simulink model "FinalProject"  (R2022b)
settings: Solver=VariableStepAuto  StartTime=0.0  StopTime=800  RelTol=1e-3
InitFcn:
  | vehicle_longitudinal_para
values from neighbouring files (symbols this model uses):
  A = [-1/(R2*C2), 0; 0, 0]    [vehicle_longitudinal_para.m]
  ai = [0.0059 0.0049 0.0039 0.0028 0.0036 0.006 0.0082 0.008 0.009 0.0099]    [vehicle_longitudinal_para.m]
  B = [1/C2; ni/Cn]    [vehicle_longitudinal_para.m]
  BatteryCapacity = 10080    [vehicle_longitudinal_para.m]
  bi = [3.5052 3.5188 3.5397 3.5728 3.5416 3.4199 3.2864 3.3004 3.2232 3.1364]    [vehicle_longitudinal_para.m]
  bp = [0.05 0.15 0.25 0.35 0.45 0.55 0.65 0.75 0.85 0.95]    [vehicle_longitudinal_para.m]
  capacity = 84    [vehicle_longitudinal_para.m]
  Cr = 0.0085    [VehicleLongtitudinalModel.m]    (also in vehicle_longitudinal_para.m = 0.009)
  D = R1    (= 0.0027)    [vehicle_longitudinal_para.m]
  eng_consum_fuel = [0 0 0 0 0 0 0 0 0 0 0 0 ... (1220 elements, 61x20)]    [eng_consum_fuel.mat]    (also in vehicle_longitudinal_para.m = eng_consum_fuel * 6)
  eng_consum_spd = [52.35 55 57.6 60.2 62.85 65.45 68.05 70.7 73.3 75.9 78.55 81.15 ... (61 elements, 1x61)]    [eng_consum_fuel.mat]    (also in vehicle_longitudinal_para.m = eng_consum_spd / 2)
  eng_consum_trq = [0 137.659783677 206.489675516 275.319567355 344.149459194 412.979351032 481.809242871 550.63913471 619.469026549 688.298918387 757.128810226 825.958702065 ... (20 elements, 1x20)]    [eng_consum_fuel.mat]    (also in vehicle_longitudinal_para.m = eng_consum_trq * (1400 / 1.356 / 75))
  FD_ratio = 4.56    [vehicle_longitudinal_para.m]
  g = 9.81    [VehicleLongtitudinalModel.m]    (also in vehicle_longitudinal_para.m)
  m_map_spd = [0 52.3598775598 104.71975512 157.079632679 209.439510239 261.799387799 314.159265359 366.519142919 418.879020479 471.238898038 628.318530718]    [m_eff_map.mat]    (also in vehicle_longitudinal_para.m = [0 500 1000 1500 2000 2500 3000 3500 4000 4500 6000]*(2*pi)/)
  m_max_trq = interp1(m_spd_data,m_max_trq_data,m_map_spd,'linear')    [vehicle_longitudinal_para.m]
  P_demand = [0 22222.2222222 44444.4444444 66666.6666667 88888.8888889 111111.111111 133333.333333 155555.555556 177777.777778 200000]    [ecms_lookup.mat]    (also in ecms_model.m = linspace(0,Pmax,10); vehicle_longitudinal_para.m = linspace(0,Pmax,10))
  P_eng_opt = [0 0 0 0 0 0 0 0 0 0 0 0 ... (1100 elements, 10x10x11)]    [ecms_lookup.mat]    (also in ecms_model.m = zeros(length(P_demand),length(V_range),length(SOC_range)); vehicle_longitudinal_para.m = zeros(length(P_demand),length(V_range),length(SOC_range)))
  R_tire = 0.5    [VehicleLongtitudinalModel.m]    (also in vehicle_longitudinal_para.m = 0.74)
  SOC = [0 20 40 60 80 100]    [vehicle_longitudinal_para.m]
  SOC_H = 1.0    (= 1)    [ecms_model.m]    (also in vehicle_longitudinal_para.m = 0.9)
  SOC_L = 0.2    [ecms_model.m]    (also in vehicle_longitudinal_para.m = 0.1)
  SOC_range = [0 0.1 0.2 0.3 0.4 0.5 0.6 0.7 0.8 0.9 1]    [ecms_lookup.mat]    (also in ecms_model.m = 0:.1:1; vehicle_longitudinal_para.m = 0:.1:1)
  Speed = cdata{2}    [vehicle_longitudinal_para.m]
  testTime = [0, 1, 2, 3, 4, 5, 6, 7, 8, 9]    [vehicle_longitudinal_para.m]
  Time = cdata{1}    [vehicle_longitudinal_para.m]
  V_range = [0 23.2710566933 46.5421133865 69.8131700798 93.084226773 116.355283466 139.62634016 162.897396853 186.168453546 209.439510239]    [ecms_lookup.mat]    (also in ecms_model.m = linspace(0,Vmax,10)*2*pi/60; vehicle_longitudinal_para.m = linspace(0,Vmax,10)*2*pi/60)
  Vehicle_mass = 15076    [VehicleLongtitudinalModel.m]    (also in vehicle_longitudinal_para.m = 6273)
  weightfactor = [1 1 1 1 1 0]    [vehicle_longitudinal_para.m]
  weightfactor_ws = [0.01 0.01 1 1 1]    [vehicle_longitudinal_para.m]
  WheelSpeed = [0 30 100 150 201]    [vehicle_longitudinal_para.m]
libraries: slpidlib x2
settings Model: Creator=12159  LastModifiedBy=12159
settings SolverCC: ZeroCrossAlgorithm=Adaptive
settings DebuggingCC: IgnoredZcDiagnostic=none

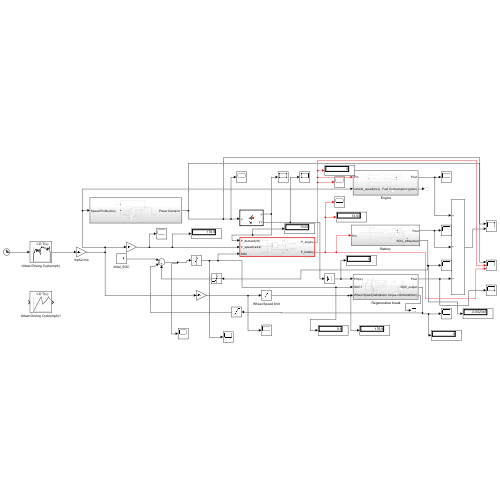
[thumbnail: Simulink's stored preview of the top-level diagram]
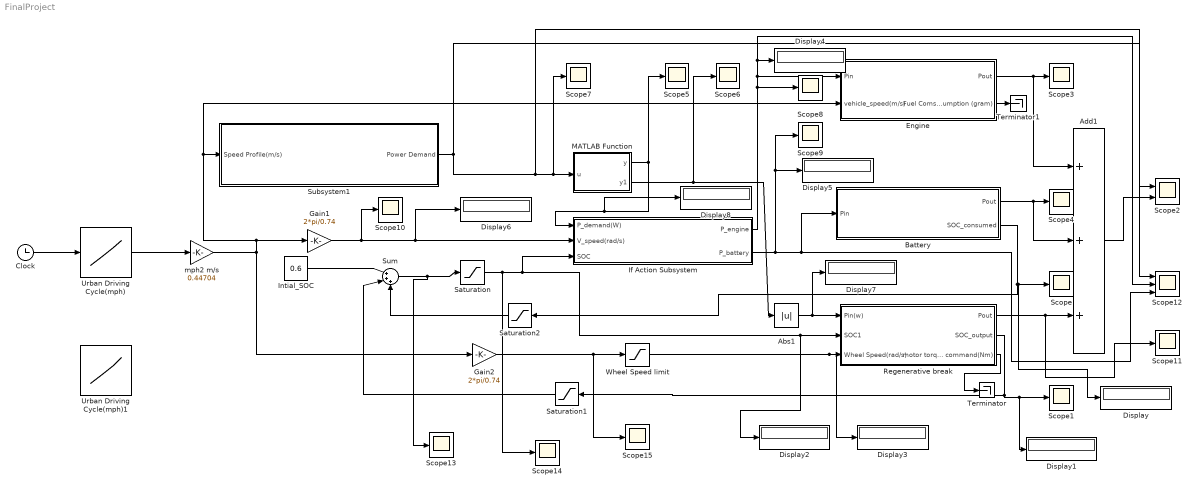
== system FinalProject ==
  " Engine" : Subsystem
  " Regenerative break" : Subsystem
  Abs1 : Abs  SaturateOnIntegerOverflow=off
  Add1 : Sum  Inputs=3
  Battery : Subsystem
  Clock : Clock
  Display{,1..8} (9 alike) : Display
  Gain1 : Gain  Gain=2*pi/0.74
  Gain2 : Gain  Gain=2*pi/0.74
  If Action Subsystem : Subsystem  TreatAsAtomicUnit=on
  Intial_SOC : Constant  Value=0.6
  MATLAB Function : MATLAB Function  TreatAsAtomicUnit=on
  Saturation : Saturate  UpperLimit=SOC_H  LowerLimit=SOC_L
  Saturation1 : Saturate  UpperLimit=SOC_H  LowerLimit=SOC_L
  Saturation2 : Saturate  UpperLimit=SOC_H  LowerLimit=SOC_L
  Scope{,1,3..11,13..15} (14 alike) : Scope
  Scope12 : Scope  NumInputPorts=3
  Scope2 : Scope  NumInputPorts=2
  Subsystem1 : Subsystem
  Sum : Sum  Inputs=|+++
  Terminator : Terminator
  Terminator1 : Terminator
  Urban Driving Cycle(mph) : Lookup_n-D  NumberOfTableDimensions=1  BreakpointsForDimension1=Time  Table=Speed  InternalRulePriority=Speed  RndMeth=Simplest
  Urban Driving Cycle(mph)1 : Lookup_n-D  NumberOfTableDimensions=1  BreakpointsForDimension1=testTime  Table=[0 10 20 30 40 20 25 30 40 32]  InternalRulePriority=Speed  RndMeth=Simplest
  Wheel Speed limit : Saturate  UpperLimit=210  LowerLimit=0.01
  mph2 m/s : Gain  Gain=0.44704
  wires:
  " Engine"/1(Pout) -> Scope3/1, Add1/1
  " Regenerative break"/1(Pout) -> Scope11/1, Add1/3
  Intial_SOC/1 -> Sum/1
  " Regenerative break"/2(SOC_output) -> Display1/1, Scope1/1, Saturation1/1
  Sum/1 -> Scope13/1, Saturation/1
  " Regenerative break"/3(motor torque command(Nm)) -> Terminator/1
  mph2 m/s/1 -> Gain1/1, Subsystem1/1(Speed Profile(m/s)), " Engine"/2(vehicle_speed(m/s)), Gain2/1
  Gain2/1 -> Wheel Speed limit/1, Scope15/1
  " Engine"/2(Fuel Comsumption (gram)) -> Terminator1/1
  Battery/1(Pout) -> Scope4/1, Add1/2
  If Action Subsystem/2(P_battery) -> Scope9/1, Display5/1, Scope12/3, Battery/1(Pin)
  Battery/2(SOC_consumed) -> Saturation2/1, Scope/1, Display/1
  Saturation/1 -> Display2/1, " Regenerative break"/2(SOC1), If Action Subsystem/3(SOC), Scope14/1
  Add1/1 -> Scope2/2
  Abs1/1 -> " Regenerative break"/1(Pin(w)), Display7/1
  MATLAB Function/1(y) -> Display8/1, If Action Subsystem/1(P_demand(W)), Scope5/1
  MATLAB Function/2(y1) -> Abs1/1, Scope6/1
  If Action Subsystem/1(P_engine) -> Scope12/2, Display4/1, " Engine"/1(Pin), Scope8/1
  Wheel Speed limit/1 -> Display3/1, " Regenerative break"/3(Wheel Speed(rad/s))
  Subsystem1/1("Power Demand ") -> Scope12/1, Scope7/1, MATLAB Function/1(u), Scope2/1
  Gain1/1 -> Scope10/1, If Action Subsystem/2(V_speed(rad/s)), Display6/1
  Clock/1 -> Urban Driving Cycle(mph)/1
  Urban Driving Cycle(mph)/1 -> mph2 m/s/1
  Saturation1/1 -> Sum/2
  Saturation2/1 -> Sum/3

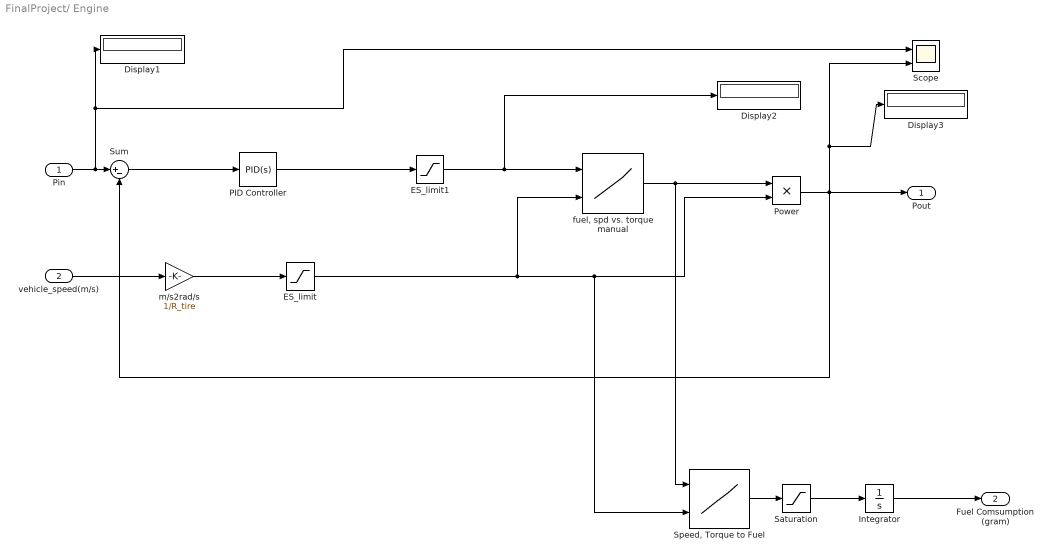
== system FinalProject/ Engine ==
  Pin : Inport
  vehicle_speed(m/s) : Inport  Port=2
  Display1 : Display
  Display2 : Display
  Display3 : Display
  ES_limit : Saturate  UpperLimit=210  LowerLimit=0
  ES_limit1 : Saturate  UpperLimit=1  LowerLimit=0
  Integrator : Integrator
  PID Controller : slpidlib/PID Controller  Controller=PID  Form=Parallel  TimeDomain=Continuous-time  UseExternalTs=off  SampleTime=-1  IntegratorMethod=Forward Euler  FilterMethod=Forward Euler  ControllerParametersSource=internal  P=1  I=1  UseKiTs=off  D=0  N=100  UseFilter=on  TunerSelectOption=Transfer Function Based (PID Tuner App)  InitialConditionSource=internal  InitialConditionForIntegrator=0  InitialConditionForFilter=0  DifferentiatorICPrevScaledInput=0  ExternalReset=none  TrackingMode=off  Kt=1  LimitOutput=off  SatLimitsSource=internal  UpperSaturationLimit=inf  LowerSaturationLimit=-inf  LinearizeAsGain=on  AntiWindupMode=none  Kb=1  LimitIntegrator=off  UpperIntegratorSaturationLimit=inf  LowerIntegratorSaturationLimit=-inf  POutMin=[]  POutMax=[]  IOutMin=[]  IOutMax=[]  DOutMin=[]  DOutMax=[]  NOutMin=[]  NOutMax=[]  SumOutMin=[]  SumOutMax=[]  SaturationOutMin=[]  SaturationOutMax=[]  PParamMin=[]  PParamMax=[]  IParamMin=[]  IParamMax=[]  DParamMin=[]  DParamMax=[]  NParamMin=[]  NParamMax=[]  KbParamMin=[]  KbParamMax=[]  KtParamMin=[]  KtParamMax=[]  KbOutMin=[]  KbOutMax=[]  KtOutMin=[]  KtOutMax=[]  IntegratorOutMin=[]  IntegratorOutMax=[]  FilterOutMin=[]  FilterOutMax=[]  SumI1OutMin=[]  SumI1OutMax=[]  SumI2OutMin=[]  SumI2OutMax=[]  SumI3OutMin=[]  SumI3OutMax=[]  SumI4OutMin=[]  SumI4OutMax=[]  SumDOutMin=[]  SumDOutMax=[]  DifferentiatorOutMin=[]  DifferentiatorOutMax=[]  FilterDiffOutCoefMin=[]  FilterDiffOutCoefMax=[]  ReciprocalOutMin=[]  ReciprocalOutMax=[]  SumDenOutMin=[]  SumDenOutMax=[]  SumNumOutMin=[]  SumNumOutMax=[]  DivideOutMin=[]  DivideOutMax=[]  UdiffTsProdOutMin=[]  UdiffTsProdOutMax=[]  NTsProdOutMin=[]  NTsProdOutMax=[]  UintegralTsProdOutMin=[]  UintegralTsProdOutMax=[]  UngainTsProdOutMin=[]  UngainTsProdOutMax=[]  ClampingZeroOutDataTypeStr=Inherit: Inherit via back propagation  ClampingZeroOutMin=[]  ClampingZeroOutMax=[]  FilterDenConstantOutDataTypeStr=Inherit: Inherit via back propagation  FilterDenConstantOutMin=[]  FilterDenConstantOutMax=[]  PCopyOutDataTypeStr=Inherit: Inherit via back propagation  PCopyOutMin=[]  PCopyOutMax=[]  NCopyOutDataTypeStr=Inherit: Inherit via back propagation  NCopyOutMin=[]  NCopyOutMax=[]  IntegratorContinuousStateAttributes=''  IntegratorStateMustResolveToSignalObject=off  IntegratorRTWStateStorageClass=Auto  FilterContinuousStateAttributes=''  FilterStateMustResolveToSignalObject=off  FilterRTWStateStorageClass=Auto  ParallelPVariant=InternalParameters  IdealPVariant=Disabled  IVariant=InternalParameters  DVariant=InternalParameters  IntegratorVariant=Continuous  SatVariant=Disabled  AWVariant=Passthrough  PCopyVariant=Disabled  TRVariant=Disabled  FdbkBlocksVariant=Forward  IdealPFdbkVariant=Disabled  SatFdbkVariant=Disabled  DerivativeFilterVariant=ContFilter  NVariant=InternalParameters  NCopyVariant=Disabled  FilterICVariant=InternalICsFilter  IntegratorICVariant=InternalICs  ExternalResetVariant=Disabled  TRSumVariant=Passthrough  SumFdbkVariant=Disabled  SumVariant=Sum_PID  TsampFilterVariant=InternalTs  TsampNgainVariant=Passthrough  TsampIntegralVariant=Passthrough  ExternalSaturationOutDataTypeStr=Inherit: Same as second input
  Power : Product
  Saturation : Saturate  UpperLimit=Inf  LowerLimit=0
  Scope : Scope  NumInputPorts=2
  "Speed, Torque to Fuel" : Lookup_n-D  BreakpointsForDimension1=eng_consum_spd  BreakpointsForDimension2=eng_consum_trq  Table=eng_consum_fuel  InternalRulePriority=Speed  RndMeth=Simplest
      settings: InputPortMap=u0,u1
  Sum : Sum  Inputs=|+-
  "fuel, spd vs. torque manual" : Lookup_n-D  BreakpointsForDimension1=[0 0.1 0.2 0.3 0.4 0.5 0.6 0.7 0.8 0.9 1]  BreakpointsForDimension2=[52.35 55 57.6 60.2 62.85 65.45 68.05 70.7 73.3 75.9 78.55 81.15 83.8 86.4 89 91.65 94.25 96.85 99.5 102.1 104.7 107.35 109.95 112.55 115.2 117.8 120.45 123.05 125.65 128.3 130.9 133.5 136.15 138.75 141.35 144 146.6 149.25 151.85 154.45 157.1 159.7 162.3 164.95 167.55 170.15 172.8 175.4 178 180.65 183.25 185.9 188.5 191.1 193.75 196.35 198.95 201.6 204.2 206.8 209.45]  Table=[0 0 0 0 0 0 0 0 0 0 0 0 0 0 0 0 0 0 0 0 0 0 0 0 0 0 0 0 0 0 0 0 0 0 0 0 0 0 0 0 0 0 0 0 0 0 0 0 0 0 0 0 0 0 0 0 0 0 0 0 0;106.452310717797 107.649950835792 108.847590953786 110.04523107178 111.242871189774 112.440511307768 113.362831858407 114.051130776794 114.739429695182 115.427728613569 116.116027531957 116.776794493609 117.286135693215 117.80924287119 118.318584070796 118.827925270403 119.351032448378 119.942969518191 120.589970501475 121.250737463127 121.897738446411 122.544739429695 123.164208456244 123.604719764012 124.04523107178 124.485742379548 124.940019665683 125.380530973451 125.821042281219 126.275319567355 126.715830875123 127.170108161259 127.610619469027 128.064896755162 128.50540806293 128.945919370698 129.386430678466 129.840707964602 130.28121927237 130.721730580138 131.176007866273 131.616519174041 132.057030481809 132.511307767945 132.951819075713 133.392330383481 133.832841691249 134.287118977384 134.727630285152 135.16814159292 135.622418879056 136.062930186824 136.51720747296 136.957718780728 137.398230088496 137.935103244838 138.34808259587 138.89872173058 139.44936086529 140 140.412979351032;212.904621435595 215.299901671583 217.695181907571 220.09046214356 222.485742379548 224.881022615536 226.725663716814 228.102261553589 229.478859390364 230.855457227139 232.232055063913 233.553588987217 234.572271386431 235.61848574238 236.637168141593 237.655850540806 238.702064896755 239.885939036382 241.17994100295 242.501474926254 243.795476892822 245.08947885939 246.328416912488 247.209439528024 248.09046214356 248.971484759095 249.880039331367 250.761061946903 251.642084562439 252.55063913471 253.431661750246 254.340216322517 255.221238938053 256.129793510324 257.01081612586 257.891838741396 258.772861356932 259.681415929204 260.562438544739 261.443461160275 262.352015732547 263.233038348083 264.114060963618 265.02261553589 265.903638151426 266.784660766962 267.665683382498 268.574237954769 269.455260570305 270.336283185841 271.244837758112 272.125860373648 273.034414945919 273.915437561455 274.796460176991 275.870206489676 276.69616519174 277.79744346116 278.89872173058 280 280.825958702065;319.356932153392 322.949852507375 326.542772861357 330.135693215339 333.728613569322 337.321533923304 340.088495575221 342.153392330383 344.218289085546 346.283185840708 348.34808259587 350.330383480826 351.858407079646 353.427728613569 354.955752212389 356.483775811209 358.053097345133 359.828908554572 361.769911504425 363.75221238938 365.693215339233 367.634218289085 369.492625368732 370.814159292035 372.135693215339 373.457227138643 374.82005899705 376.141592920354 377.463126843658 378.825958702065 380.147492625369 381.510324483776 382.83185840708 384.194690265487 385.516224188791 386.837758112094 388.159292035398 389.522123893805 390.843657817109 392.165191740413 393.52802359882 394.849557522124 396.171091445428 397.533923303835 398.855457227139 400.176991150442 401.498525073746 402.861356932153 404.182890855457 405.504424778761 406.867256637168 408.188790560472 409.551622418879 410.873156342183 412.194690265487 413.805309734513 415.044247787611 416.69616519174 418.34808259587 420 421.238938053097;425.80924287119 430.599803343166 435.390363815143 440.180924287119 444.971484759095 449.762045231072 453.451327433628 456.204523107178 458.957718780728 461.710914454277 464.464110127827 467.107177974435 469.144542772861 471.236971484759 473.274336283186 475.311701081613 477.40412979351 479.771878072763 482.3598820059 485.002949852507 487.590953785644 490.178957718781 492.656833824975 494.418879056047 496.180924287119 497.942969518191 499.760078662734 501.522123893805 503.284169124877 505.10127826942 506.863323500492 508.680432645034 510.442477876106 512.259587020649 514.021632251721 515.783677482793 517.545722713864 519.362831858407 521.124877089479 522.886922320551 524.704031465093 526.466076696165 528.228121927237 530.04523107178 531.807276302852 533.569321533923 535.331366764995 537.148475909538 538.91052114061 ...(+6299 chars)]  InternalRulePriority=Speed  RndMeth=Simplest
      settings: InputPortMap=u0,u1
  m/s2rad/s : Gain  Gain=1/R_tire
  Pout : Outport
  Fuel Comsumption (gram) : Outport  Port=2
  wires:
  vehicle_speed(m/s)/1 -> m/s2rad/s/1
  Power/1 -> Pout/1, Scope/2, Display3/1, Sum/2
  "fuel, spd vs. torque manual"/1 -> "Speed, Torque to Fuel"/1, Power/1
  ES_limit/1 -> "fuel, spd vs. torque manual"/2, "Speed, Torque to Fuel"/2, Power/2
  Pin/1 -> Scope/1, Display1/1, Sum/1
  Sum/1 -> PID Controller/1
  PID Controller/1 -> ES_limit1/1
  ES_limit1/1 -> "fuel, spd vs. torque manual"/1, Display2/1
  m/s2rad/s/1 -> ES_limit/1
  "Speed, Torque to Fuel"/1 -> Saturation/1
  Integrator/1 -> Fuel Comsumption (gram)/1
  Saturation/1 -> Integrator/1

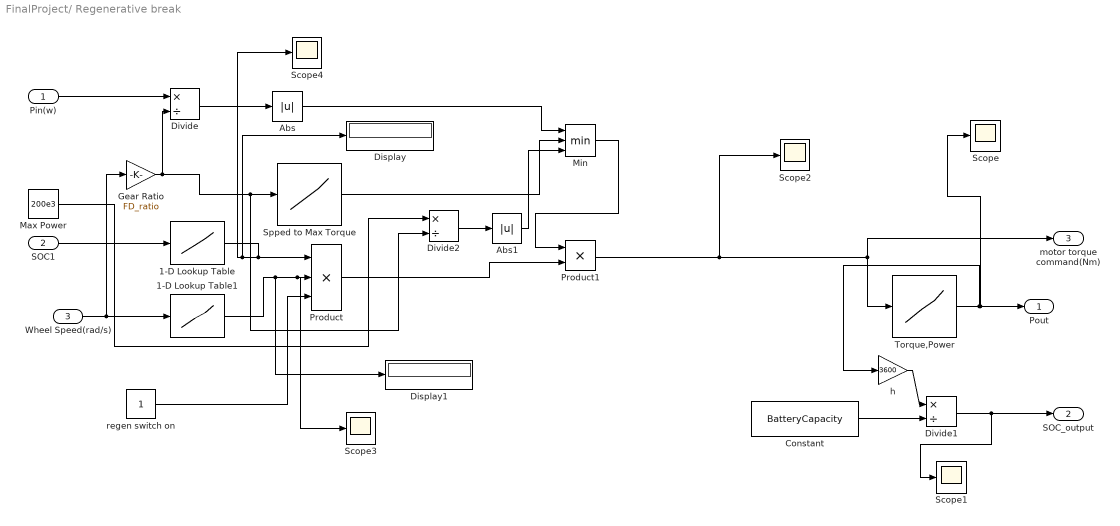
== system FinalProject/ Regenerative break ==
  Pin(w) : Inport
  SOC1 : Inport  Port=2
  Wheel Speed(rad/s) : Inport  Port=3
  1-D Lookup Table : Lookup_n-D  NumberOfTableDimensions=1  BreakpointsForDimension1=SOC  Table=weightfactor  InternalRulePriority=Speed  RndMeth=Simplest
  1-D Lookup Table1 : Lookup_n-D  NumberOfTableDimensions=1  BreakpointsForDimension1=WheelSpeed  Table=weightfactor_ws  InternalRulePriority=Speed  RndMeth=Simplest
  Abs : Abs  SaturateOnIntegerOverflow=off
  Abs1 : Abs  SaturateOnIntegerOverflow=off
  Constant : Constant  Value=BatteryCapacity
  Display : Display
  Display1 : Display
  Divide : Product  Inputs=*/
  Divide1 : Product  Inputs=*/
  Divide2 : Product  Inputs=*/
  Gear Ratio : Gain  Gain=FD_ratio
  Max Power : Constant  Value=200e3
  Min : MinMax  Inputs=3
  Product : Product  Inputs=3
  Product1 : Product
  Scope{,1..4} (5 alike) : Scope
  Spped to Max Torque : Lookup_n-D  NumberOfTableDimensions=1  BreakpointsForDimension1=m_map_spd  Table=m_max_trq  InternalRulePriority=Speed  RndMeth=Simplest
  Torque,Power : Lookup_n-D  NumberOfTableDimensions=1  BreakpointsForDimension1=[0 3000]  Table=[0 200000]  InternalRulePriority=Speed  RndMeth=Simplest
  h : Gain  Gain=3600
  regen switch on : Constant
  Pout : Outport
  SOC_output : Outport  Port=2
  motor torque command(Nm) : Outport  Port=3
  wires:
  Wheel Speed(rad/s)/1 -> 1-D Lookup Table1/1, Gear Ratio/1
  1-D Lookup Table/1 -> Display/1, Scope4/1, Product/1
  regen switch on/1 -> Product/3
  Pin(w)/1 -> Divide/1
  Product1/1 -> Scope2/1, Torque,Power/1, motor torque command(Nm)/1
  Product/1 -> Product1/2
  SOC1/1 -> 1-D Lookup Table/1
  Abs/1 -> Min/1
  1-D Lookup Table1/1 -> Display1/1, Scope3/1, Product/2
  Divide/1 -> Abs/1
  Torque,Power/1 -> h/1, Scope/1, Pout/1
  h/1 -> Divide1/1
  Constant/1 -> Divide1/2
  Divide1/1 -> Scope1/1, SOC_output/1
  Gear Ratio/1 -> Spped to Max Torque/1, Divide2/2, Divide/2
  Spped to Max Torque/1 -> Min/2
  Max Power/1 -> Divide2/1
  Divide2/1 -> Abs1/1
  Abs1/1 -> Min/3
  Min/1 -> Product1/1

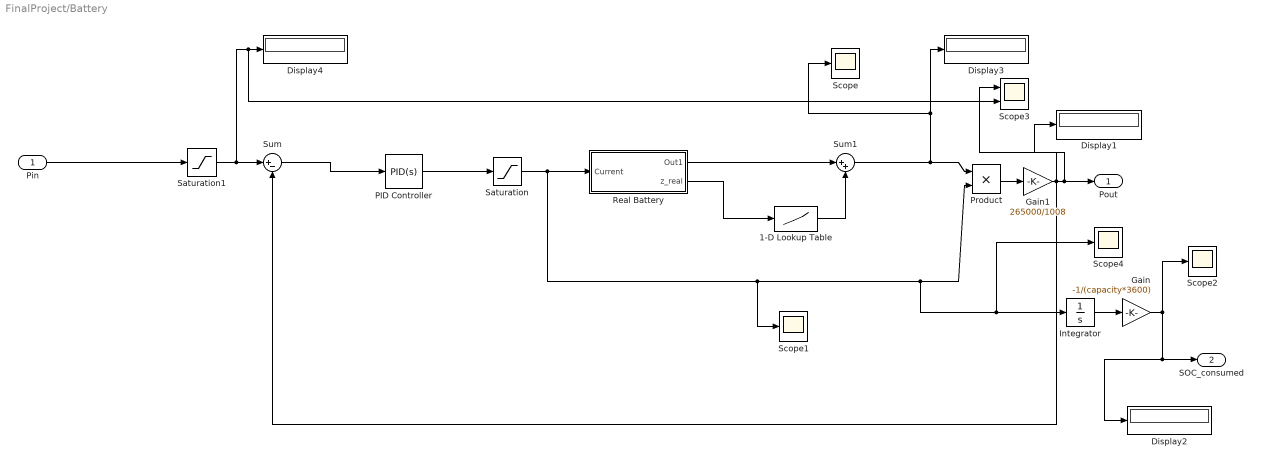
== system FinalProject/Battery ==
  Pin : Inport
  1-D Lookup Table : Lookup_n-D  NumberOfTableDimensions=1  BreakpointsForDimension1=bp  Table=bi  InternalRulePriority=Speed  RndMeth=Simplest
  Display{1..4} (4 alike) : Display
  Gain : Gain  Gain=-1/(capacity*3600)
  Gain1 : Gain  Gain=265000/1008
  Integrator : Integrator
  PID Controller : slpidlib/PID Controller  Controller=PID  Form=Parallel  TimeDomain=Continuous-time  UseExternalTs=off  SampleTime=-1  IntegratorMethod=Forward Euler  FilterMethod=Forward Euler  ControllerParametersSource=internal  P=12  I=1  UseKiTs=off  D=0  N=100  UseFilter=on  TunerSelectOption=Transfer Function Based (PID Tuner App)  InitialConditionSource=internal  InitialConditionForIntegrator=0  InitialConditionForFilter=0  DifferentiatorICPrevScaledInput=0  ExternalReset=none  TrackingMode=off  Kt=1  LimitOutput=off  SatLimitsSource=internal  UpperSaturationLimit=inf  LowerSaturationLimit=-inf  LinearizeAsGain=on  AntiWindupMode=none  Kb=1  LimitIntegrator=off  UpperIntegratorSaturationLimit=inf  LowerIntegratorSaturationLimit=-inf  POutMin=[]  POutMax=[]  IOutMin=[]  IOutMax=[]  DOutMin=[]  DOutMax=[]  NOutMin=[]  NOutMax=[]  SumOutMin=[]  SumOutMax=[]  SaturationOutMin=[]  SaturationOutMax=[]  PParamMin=[]  PParamMax=[]  IParamMin=[]  IParamMax=[]  DParamMin=[]  DParamMax=[]  NParamMin=[]  NParamMax=[]  KbParamMin=[]  KbParamMax=[]  KtParamMin=[]  KtParamMax=[]  KbOutMin=[]  KbOutMax=[]  KtOutMin=[]  KtOutMax=[]  IntegratorOutMin=[]  IntegratorOutMax=[]  FilterOutMin=[]  FilterOutMax=[]  SumI1OutMin=[]  SumI1OutMax=[]  SumI2OutMin=[]  SumI2OutMax=[]  SumI3OutMin=[]  SumI3OutMax=[]  SumI4OutMin=[]  SumI4OutMax=[]  SumDOutMin=[]  SumDOutMax=[]  DifferentiatorOutMin=[]  DifferentiatorOutMax=[]  FilterDiffOutCoefMin=[]  FilterDiffOutCoefMax=[]  ReciprocalOutMin=[]  ReciprocalOutMax=[]  SumDenOutMin=[]  SumDenOutMax=[]  SumNumOutMin=[]  SumNumOutMax=[]  DivideOutMin=[]  DivideOutMax=[]  UdiffTsProdOutMin=[]  UdiffTsProdOutMax=[]  NTsProdOutMin=[]  NTsProdOutMax=[]  UintegralTsProdOutMin=[]  UintegralTsProdOutMax=[]  UngainTsProdOutMin=[]  UngainTsProdOutMax=[]  ClampingZeroOutDataTypeStr=Inherit: Inherit via back propagation  ClampingZeroOutMin=[]  ClampingZeroOutMax=[]  FilterDenConstantOutDataTypeStr=Inherit: Inherit via back propagation  FilterDenConstantOutMin=[]  FilterDenConstantOutMax=[]  PCopyOutDataTypeStr=Inherit: Inherit via back propagation  PCopyOutMin=[]  PCopyOutMax=[]  NCopyOutDataTypeStr=Inherit: Inherit via back propagation  NCopyOutMin=[]  NCopyOutMax=[]  IntegratorContinuousStateAttributes=''  IntegratorStateMustResolveToSignalObject=off  IntegratorRTWStateStorageClass=Auto  FilterContinuousStateAttributes=''  FilterStateMustResolveToSignalObject=off  FilterRTWStateStorageClass=Auto  ParallelPVariant=InternalParameters  IdealPVariant=Disabled  IVariant=InternalParameters  DVariant=InternalParameters  IntegratorVariant=Continuous  SatVariant=Disabled  AWVariant=Passthrough  PCopyVariant=Disabled  TRVariant=Disabled  FdbkBlocksVariant=Forward  IdealPFdbkVariant=Disabled  SatFdbkVariant=Disabled  DerivativeFilterVariant=ContFilter  NVariant=InternalParameters  NCopyVariant=Disabled  FilterICVariant=InternalICsFilter  IntegratorICVariant=InternalICs  ExternalResetVariant=Disabled  TRSumVariant=Passthrough  SumFdbkVariant=Disabled  SumVariant=Sum_PID  TsampFilterVariant=InternalTs  TsampNgainVariant=Passthrough  TsampIntegralVariant=Passthrough  ExternalSaturationOutDataTypeStr=Inherit: Same as second input
  Product : Product
  Real Battery : Subsystem
  Saturation : Saturate  UpperLimit=84  LowerLimit=0
  Saturation1 : Saturate  UpperLimit=inf  LowerLimit=0
  Scope{,1..2,4} (4 alike) : Scope
  Scope3 : Scope  NumInputPorts=2
  Sum : Sum  Inputs=|+-
  Sum1 : Sum  Inputs=|++
  Pout : Outport
  SOC_consumed : Outport  Port=2
  wires:
  1-D Lookup Table/1 -> Sum1/2
  Real Battery/2(z_real) -> 1-D Lookup Table/1
  Real Battery/1(Out1) -> Sum1/1
  PID Controller/1 -> Saturation/1
  Sum/1 -> PID Controller/1
  Integrator/1 -> Gain/1
  Gain/1 -> Scope2/1, Display2/1, SOC_consumed/1
  Saturation/1 -> Product/2, Scope4/1, Integrator/1, Scope1/1, Real Battery/1(Current)
  Saturation1/1 -> Sum/1, Scope3/2, Display4/1
  Sum1/1 -> Product/1, Scope/1, Display3/1
  Pin/1 -> Saturation1/1
  Product/1 -> Gain1/1
  Gain1/1 -> Pout/1, Display1/1, Sum/2, Scope3/1

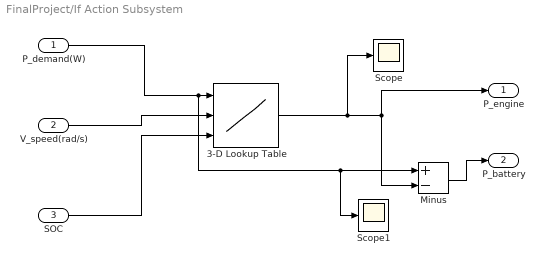
== system FinalProject/If Action Subsystem ==
  P_demand(W) : Inport
  V_speed(rad/s) : Inport  Port=2
  SOC : Inport  Port=3
  3-D Lookup Table : Lookup_n-D  NumberOfTableDimensions=3  BreakpointsForDimension1=P_demand  BreakpointsForDimension2=V_range  BreakpointsForDimension3=SOC_range  Table=P_eng_opt  InternalRulePriority=Speed  RndMeth=Simplest
      settings: InputPortMap=u0,u1,u2
  Minus : Sum  Inputs=+-
  Scope : Scope
  Scope1 : Scope
  P_engine : Outport
  P_battery : Outport  Port=2
  wires:
  3-D Lookup Table/1 -> Scope/1, Minus/2, P_engine/1
  SOC/1 -> 3-D Lookup Table/3
  V_speed(rad/s)/1 -> 3-D Lookup Table/2
  Minus/1 -> P_battery/1
  P_demand(W)/1 -> Scope1/1, Minus/1, 3-D Lookup Table/1

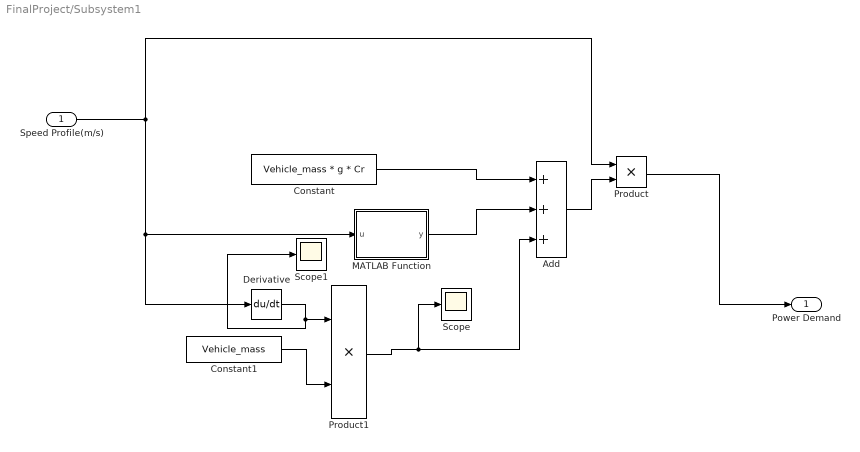
== system FinalProject/Subsystem1 ==
  Speed Profile(m/s) : Inport
  Add : Sum  Inputs=+++
  Constant : Constant  Value=Vehicle_mass * g * Cr
  Constant1 : Constant  Value=Vehicle_mass
  Derivative : Derivative
  MATLAB Function : MATLAB Function  TreatAsAtomicUnit=on
  Product : Product
  Product1 : Product
  Scope : Scope
  Scope1 : Scope
  "Power Demand " : Outport
  wires:
  Add/1 -> Product/2
  Speed Profile(m/s)/1 -> Derivative/1, MATLAB Function/1(u), Product/1
  MATLAB Function/1(y) -> Add/2
  Constant/1 -> Add/1
  Derivative/1 -> Scope1/1, Product1/1
  Constant1/1 -> Product1/2
  Product1/1 -> Scope/1, Add/3
  Product/1 -> "Power Demand "/1

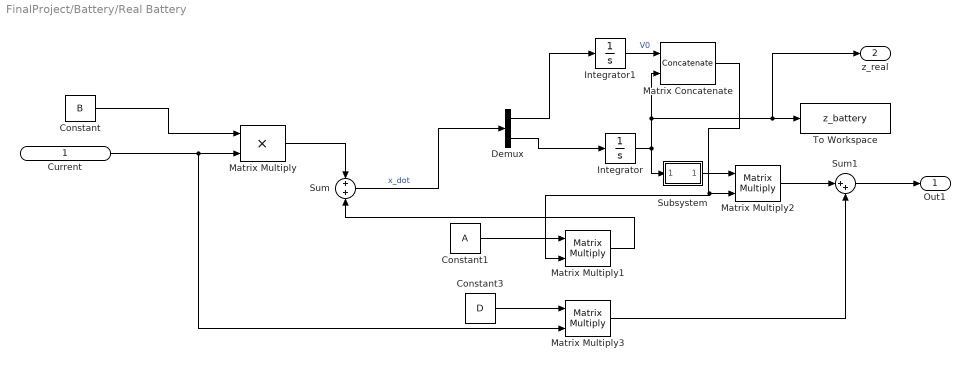
== system FinalProject/Battery/Real Battery ==
  Current : Inport
  Constant : Constant  Value=B  VectorParams1D=off
  Constant1 : Constant  Value=A
  Constant3 : Constant  Value=D  VectorParams1D=off
  Demux : Demux  Outputs=2
  Integrator : Integrator  InitialCondition=.5  LimitOutput=on  UpperSaturationLimit=1  LowerSaturationLimit=0
  Integrator1 : Integrator  InitialCondition=3.7
  Matrix Concatenate : Concatenate  Mode=Multidimensional array
  Matrix Multiply : Product
  Matrix Multiply1 : Product  Multiplication=Matrix(*)
  Matrix Multiply2 : Product  Multiplication=Matrix(*)
  Matrix Multiply3 : Product  Multiplication=Matrix(*)
  Subsystem : Subsystem
  Sum : Sum
  Sum1 : Sum  Inputs=|++
  To Workspace : ToWorkspace  VariableName=z_battery  SaveFormat=Timeseries  SampleTime=-1
  Out1 : Outport
  z_real : Outport  Port=2
  wires:
  Sum/1 -> Demux/1  "x_dot"
  Current/1 -> Matrix Multiply3/2, Matrix Multiply/2
  Matrix Multiply1/1 -> Sum/2
  Matrix Multiply2/1 -> Sum1/1
  Matrix Multiply3/1 -> Sum1/2
  Sum1/1 -> Out1/1
  Matrix Multiply/1 -> Sum/1
  Constant1/1 -> Matrix Multiply1/1
  Matrix Concatenate/1 -> Matrix Multiply1/2, Matrix Multiply2/2
  Demux/2 -> Integrator/1
  Integrator/1 -> Subsystem/1(Input), z_real/1, To Workspace/1, Matrix Concatenate/2
  Integrator1/1 -> Matrix Concatenate/1  "V0"
  Constant3/1 -> Matrix Multiply3/1
  Constant/1 -> Matrix Multiply/1
  Demux/1 -> Integrator1/1
  Subsystem/1(Out1) -> Matrix Multiply2/1

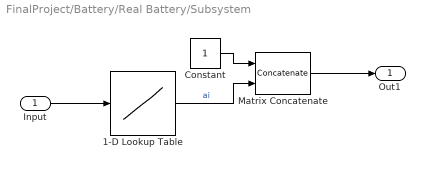
== system FinalProject/Battery/Real Battery/Subsystem ==
  Input : Inport
  1-D Lookup Table : Lookup_n-D  NumberOfTableDimensions=1  BreakpointsForDimension1=bp  Table=ai  InternalRulePriority=Speed  RndMeth=Simplest
  Constant : Constant  VectorParams1D=off
  Matrix Concatenate : Concatenate  Mode=Multidimensional array  ConcatenateDimension=2
  Out1 : Outport
  wires:
  Input/1 -> 1-D Lookup Table/1
  1-D Lookup Table/1 -> Matrix Concatenate/2  "ai"
  Matrix Concatenate/1 -> Out1/1
  Constant/1 -> Matrix Concatenate/1

== matlab function FinalProject/MATLAB Function ==
  data: u input; y output; y1 output
function [y,y1] = fcn(u)
if u > 0
    y = u;
    y1 = 0;
else
    y1 = u;
    y = 0;
end

== matlab function FinalProject/Subsystem1/MATLAB Function ==
  data: u input; y output
function y = fcn(u)
Vehicle_mass = 15076; % vehicle total mass, kg
g = 9.81; % Gravity constant
Cr = 0.0085; % Rolling resistance constant
%R_tire = 0.5; % Radius of the tire, m

A_front = 9.5; % Area of the front, m^2
Cd = 0.7963; % Aero drag coefficient
rho_air = 1.2; % Air density kg/m^3

%FR = 1.18; % final drive gear ratio
y = 0.5*A_front*rho_air*Cd*u^2;
